simulink model "pH_completo_simulacion"  (R2015a)
settings: Solver=ode45  StartTime=0.0  StopTime=inf  RelTol=1e-3
undefined symbols (not defined in the file or in its folder): Ki, Kp
libraries: instrumentlib x2, simulink x1
settings Model: Creator=Hector  LastModifiedBy=Hector
settings DebuggingCC: UnderspecifiedInitializationDetection=Classic  MergeDetectMultiDrivingBlocksExec=none  SolverPrmCheckMsg=warning  StateNameClashWarn=warning

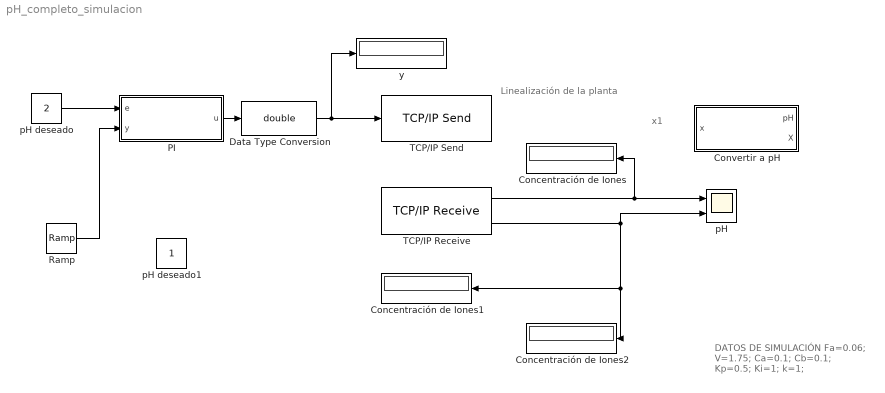
== system pH_completo_simulacion ==
  note: Linealización de la planta
  note: DATOS DE SIMULACIÓN
      | Fa=0.06;
      | V=1.75;
      | Ca=0.1;
      | Cb=0.1;
      | Kp=0.5;
      | Ki=1;
      | k=1;
  note: x1
  Concentración de Iones : Display
  Concentración de Iones1 : Display
  Concentración de Iones2 : Display
  Convertir a pH : Subsystem
  Data Type Conversion : DataTypeConversion  OutDataTypeStr=double
  PI : Subsystem
  Ramp : simulink/Sources/Ramp  slope=1  start=0  X0=0
  TCP/IP Receive : instrumentlib/TCP//IP Receive  Host=192.168.0.100  Port=80  DataSize="[1  6]"  EnableBlockingMode=off  Timeout=10  SampleTime=1  DataType=single  ByteOrder=LittleEndian
  TCP/IP Send : instrumentlib/TCP//IP Send  Host=192.168.0.100  Port=80  EnableBlockingMode=off  Timeout=10  ByteOrder=LittleEndian
  pH : Scope  NumInputPorts=2
      settings: YMin=-5~-5  YMax=5~5
  pH deseado : Constant  Value=2
  pH deseado1 : Constant
  y : Display
  wires:
  pH deseado/1 -> PI/1(e)
  TCP/IP Receive/1 -> pH/1, Concentración de Iones/1
  TCP/IP Receive/2 -> Concentración de Iones2/1, Concentración de Iones1/1, pH/2
  PI/1(u) -> Data Type Conversion/1
  Data Type Conversion/1 -> y/1, TCP/IP Send/1
  Ramp/1 -> PI/2(y)

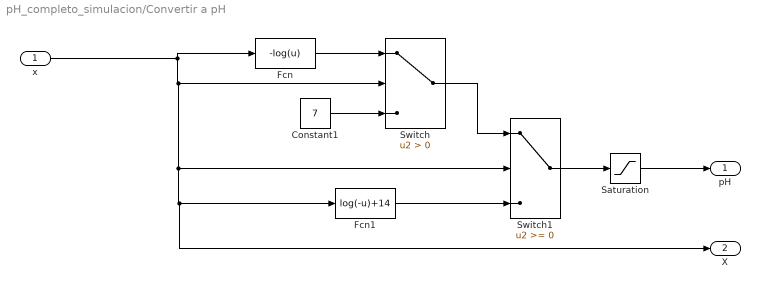
== system pH_completo_simulacion/Convertir a pH ==
  x : Inport
  Constant1 : Constant  Value=7
  Fcn : Fcn  Expr=-log(u)
  Fcn1 : Fcn  Expr=log(-u)+14
  Saturation : Saturate  UpperLimit=14  LowerLimit=0
  Switch : Switch  Criteria=u2 > Threshold
  Switch1 : Switch
  pH : Outport
  X : Outport  Port=2
  wires:
  Switch1/1 -> Saturation/1
  Switch/1 -> Switch1/1
  Constant1/1 -> Switch/3
  Fcn/1 -> Switch/1
  Fcn1/1 -> Switch1/3
  Saturation/1 -> pH/1
  x/1 -> Fcn/1, X/1, Fcn1/1, Switch1/2, Switch/2

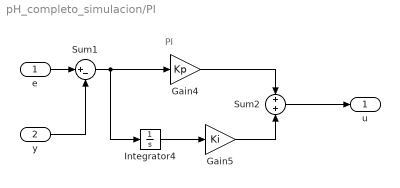
== system pH_completo_simulacion/PI ==
  note: PI
  e : Inport
  y : Inport  Port=2
  Gain4 : Gain  Gain=Kp
  Gain5 : Gain  Gain=Ki
  Integrator4 : Integrator
  Sum1 : Sum  Inputs=|+-
  Sum2 : Sum
  u : Outport
  wires:
  y/1 -> Sum1/2
  Sum1/1 -> Integrator4/1, Gain4/1
  Integrator4/1 -> Gain5/1
  Gain4/1 -> Sum2/1
  Gain5/1 -> Sum2/2
  e/1 -> Sum1/1
  Sum2/1 -> u/1
